simulink model "acc_RR_backup"  (R2021b)
settings: Solver=FixedStepAuto  StartTime=0.0  StopTime=40  FixedStep=0.0005  RelTol=1e-3
values from neighbouring files (symbols this model uses):
  s_path = [0 1.10508939428 2.2141958029 3.32141571172 4.42705301151 5.53154548532 6.63517443471 7.73808041313 8.84055018688 9.94289959674 11.0453539299 12.1480581097 ... (1001 elements, 1001x1)]    [200_100radius.mat]    (also in LV_Clothoid_S_Turn_path.mat = [0 0.966832089581 1.93621320584 2.90214024471 3.86476766313 ; NEDC_path.mat = [0 0.414605943146 0.832514087334 1.25401518562 1.68216660344; Straight_East_into_curve.mat = [0 1.65770560069 3.32192925577 4.98420060507 6.64484613518 8; acc_plot_backup.m = Station_HV_m)
  X_path = [0 1.10508939428 2.2141958029 3.32141571172 4.42705301151 5.53154548532 6.63517443471 7.73808041313 8.84055018688 9.94289959674 11.0453539299 12.1480581097 ... (1001 elements, 1001x1)]    [200_100radius.mat]    (also in LV_Clothoid_S_Turn_path.mat = [-10 -9.03316791042 -8.06378679416 -7.09785975529 -6.1352323; NEDC_path.mat = [0 0.414605943146 0.832514087334 1.25401518562 1.68216660344; Straight_East_into_curve.mat = [0 1.65770560069 3.32192925577 4.98420060507 6.64484613518 8; acc_plot_backup.m = X_HV_m)
  Y_path = [0 -1.70364610795e-18 -7.41532896709e-18 1.46822109542e-17 4.74557362791e-17 6.12980216762e-17 9.25043977736e-17 1.24088240159e-16 1.5099156923e-16 1.7058517853e-16 1.90629227614e-16 2.09673434424e-16 ... (1001 elements, 1001x1)]    [200_100radius.mat]    (also in LV_Clothoid_S_Turn_path.mat = [0 -8.46153035536e-19 5.07382551045e-18 2.07356032218e-17 3.; NEDC_path.mat = [0 -3.50680326162e-18 -2.14111304971e-18 3.38197671014e-18 3; Straight_East_into_curve.mat = [0 1.29197709199e-18 2.81882429322e-18 3.49020462564e-17 6.7; acc_plot_backup.m = Y_HV_m)
undefined symbols (not defined in the file or in its folder): C_TICK_TIME_S, ENUM_ACCSTATE_DISABLED, ENUM_ACCSTATE_OFF, ENUM_ACCSTATE_STANDBY, FALSE, KVDI_ACCLongPressTime_ms, KVDI_ACCMaxActSpeed_kph, KVDI_ACCSetSpdIntial_kph, KVDI_ACCSpdLargeChange_kph, KVDI_LongPressConTime_ms, ONE_FLOAT, ONE_INT, R, Rw, T, TRUE, ZERO_FLOAT, ZERO_INT
libraries: simulink x15, simulink_extras x2, Solver_SF x1
(part 2 of 4)

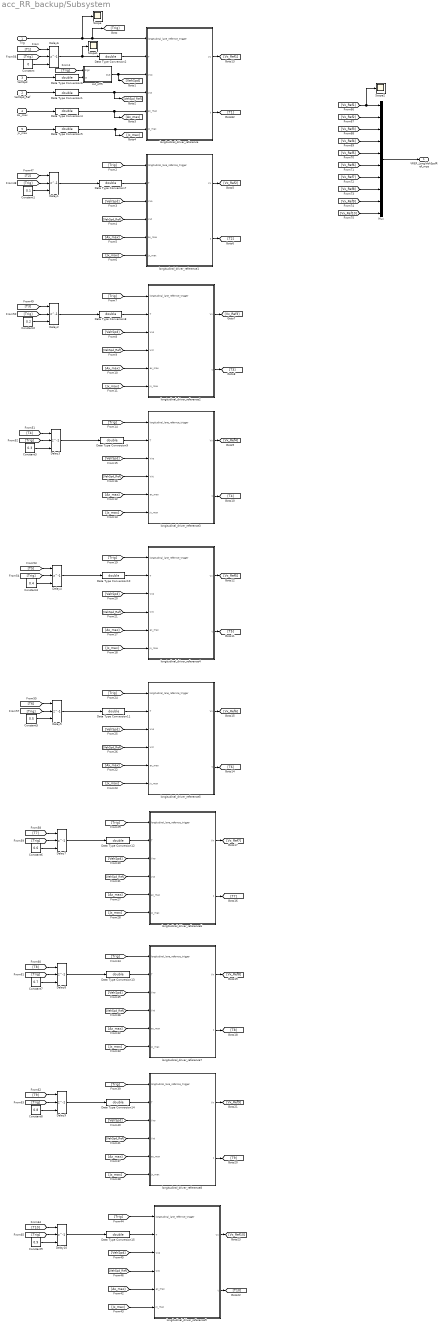
== system acc_RR_backup/Subsystem ==
  "Trig " : Inport
  VehSpd_Ref : Inport  Port=2
  VehSpd : Inport  Port=3
  Ax_max : Inport  Port=4
  Jx_max : Inport  Port=5
  Constant : Constant  Value=0
  Constant1 : Constant  Value=0.1
  Constant2 : Constant  Value=0.2
  Constant3 : Constant  Value=0.3
  Constant4 : Constant  Value=0.4
  Constant5 : Constant  Value=0.5
  Constant6 : Constant  Value=0.6
  Constant7 : Constant  Value=0.7
  Constant8 : Constant  Value=0.8
  Constant9 : Constant  Value=0.9
  Data Type Conversion{1..2,4..15} (14 alike) : DataTypeConversion  OutDataTypeStr=double
  Delay{1..10} (10 alike) : Delay  DelayLength=1  InitialConditionSource=Input port  ExternalReset=Rising
      settings: InputPortMap=u0,r5,p4
  Mux : Mux  Inputs=10
  Scope : Scope
  Scope1 : Scope
  Scope2 : Scope
  cut_off5 : Subsystem
  longitudinal_driver_reference : MATLAB Function  TreatAsAtomicUnit=on
  longitudinal_driver_reference1 : MATLAB Function  TreatAsAtomicUnit=on
  longitudinal_driver_reference2 : MATLAB Function  TreatAsAtomicUnit=on
  longitudinal_driver_reference3 : MATLAB Function  TreatAsAtomicUnit=on
  longitudinal_driver_reference4 : MATLAB Function  TreatAsAtomicUnit=on
  longitudinal_driver_reference5 : MATLAB Function  TreatAsAtomicUnit=on
  longitudinal_driver_reference6 : MATLAB Function  TreatAsAtomicUnit=on
  longitudinal_driver_reference7 : MATLAB Function  TreatAsAtomicUnit=on
  longitudinal_driver_reference8 : MATLAB Function  TreatAsAtomicUnit=on
  longitudinal_driver_reference9 : MATLAB Function  TreatAsAtomicUnit=on
  "VREF_LongiVehSpdRef_mps " : Outport
  wires:
  longitudinal_driver_reference/1(Vx) -> [Vx_Ref1]
  Mux/1 -> "VREF_LongiVehSpdRef_mps "/1
  Constant/1 -> Delay6/3
  [T1] -> Delay6/1
  Ax_max/1 -> Data Type Conversion4/1
  Jx_max/1 -> Data Type Conversion5/1
  VehSpd_Ref/1 -> Data Type Conversion1/1
  longitudinal_driver_reference/2(t) -> [T1]
  Delay6/1 -> Scope1/1, Data Type Conversion2/1
  [Trig] -> Delay6/2
  "Trig "/1 -> Scope/1, [Trig], longitudinal_driver_reference/1(longitudinal_lane_refernce_trigger)
  Data Type Conversion2/1 -> longitudinal_driver_reference/2(T)
  VehSpd/1 -> Data Type Conversion6/1
  Data Type Conversion1/1 -> [VehSpd_Ref], longitudinal_driver_reference/4(Vxt)
  cut_off5/1(Out) -> [VehSpd], longitudinal_driver_reference/3(Vxo)
  Data Type Conversion6/1 -> cut_off5/2(in)
  [Trig] -> cut_off5/1(sign)
  Data Type Conversion5/1 -> [Jx_max], longitudinal_driver_reference/6(jx_max)
  Data Type Conversion4/1 -> [Ax_max], longitudinal_driver_reference/5(ax_max)
  [Trig] -> longitudinal_driver_reference1/1(longitudinal_lane_refernce_trigger)
  [VehSpd] -> longitudinal_driver_reference1/3(Vxo)
  [VehSpd_Ref] -> longitudinal_driver_reference1/4(Vxt)
  [Ax_max] -> longitudinal_driver_reference1/5(ax_max)
  [Jx_max] -> longitudinal_driver_reference1/6(jx_max)
  [Jx_max] -> longitudinal_driver_reference2/6(jx_max)
  [Ax_max] -> longitudinal_driver_reference2/5(ax_max)
  [VehSpd_Ref] -> longitudinal_driver_reference2/4(Vxt)
  [VehSpd] -> longitudinal_driver_reference2/3(Vxo)
  [Trig] -> longitudinal_driver_reference2/1(longitudinal_lane_refernce_trigger)
  [Trig] -> longitudinal_driver_reference3/1(longitudinal_lane_refernce_trigger)
  [VehSpd] -> longitudinal_driver_reference3/3(Vxo)
  [VehSpd_Ref] -> longitudinal_driver_reference3/4(Vxt)
  [Ax_max] -> longitudinal_driver_reference3/5(ax_max)
  [Jx_max] -> longitudinal_driver_reference3/6(jx_max)
  [Jx_max] -> longitudinal_driver_reference4/6(jx_max)
  [Ax_max] -> longitudinal_driver_reference4/5(ax_max)
  [VehSpd_Ref] -> longitudinal_driver_reference4/4(Vxt)
  [VehSpd] -> longitudinal_driver_reference4/3(Vxo)
  [Trig] -> longitudinal_driver_reference4/1(longitudinal_lane_refernce_trigger)
  [Trig] -> longitudinal_driver_reference5/1(longitudinal_lane_refernce_trigger)
  [VehSpd] -> longitudinal_driver_reference5/3(Vxo)
  [VehSpd_Ref] -> longitudinal_driver_reference5/4(Vxt)
  [Ax_max] -> longitudinal_driver_reference5/5(ax_max)
  [Jx_max] -> longitudinal_driver_reference5/6(jx_max)
  [Jx_max] -> longitudinal_driver_reference6/6(jx_max)
  [Ax_max] -> longitudinal_driver_reference6/5(ax_max)
  [VehSpd_Ref] -> longitudinal_driver_reference6/4(Vxt)
  [VehSpd] -> longitudinal_driver_reference6/3(Vxo)
  [Trig] -> longitudinal_driver_reference6/1(longitudinal_lane_refernce_trigger)
  [Trig] -> longitudinal_driver_reference7/1(longitudinal_lane_refernce_trigger)
  [VehSpd] -> longitudinal_driver_reference7/3(Vxo)
  [VehSpd_Ref] -> longitudinal_driver_reference7/4(Vxt)
  [Ax_max] -> longitudinal_driver_reference7/5(ax_max)
  [Jx_max] -> longitudinal_driver_reference7/6(jx_max)
  [Jx_max] -> longitudinal_driver_reference8/6(jx_max)
  [Ax_max] -> longitudinal_driver_reference8/5(ax_max)
  [VehSpd_Ref] -> longitudinal_driver_reference8/4(Vxt)
  [VehSpd] -> longitudinal_driver_reference8/3(Vxo)
  [Trig] -> longitudinal_driver_reference8/1(longitudinal_lane_refernce_trigger)
  [Trig] -> longitudinal_driver_reference9/1(longitudinal_lane_refernce_trigger)
  [VehSpd] -> longitudinal_driver_reference9/3(Vxo)
  [VehSpd_Ref] -> longitudinal_driver_reference9/4(Vxt)
  [Ax_max] -> longitudinal_driver_reference9/5(ax_max)
  [Jx_max] -> longitudinal_driver_reference9/6(jx_max)
  longitudinal_driver_reference1/1(Vx) -> [Vx_Ref2]
  longitudinal_driver_reference1/2(t) -> [T2]
  [Trig] -> Delay1/2
  Delay1/1 -> Data Type Conversion7/1
  [T2] -> Delay1/1
  Data Type Conversion7/1 -> longitudinal_driver_reference1/2(T)
  Constant1/1 -> Delay1/3
  Constant2/1 -> Delay2/3
  Data Type Conversion8/1 -> longitudinal_driver_reference2/2(T)
  [T3] -> Delay2/1
  Delay2/1 -> Data Type Conversion8/1
  [Trig] -> Delay2/2
  longitudinal_driver_reference2/2(t) -> [T3]
  longitudinal_driver_reference2/1(Vx) -> [Vx_Ref3]
  [Trig] -> Delay3/2
  Delay3/1 -> Data Type Conversion9/1
  [T4] -> Delay3/1
  Data Type Conversion9/1 -> longitudinal_driver_reference3/2(T)
  Constant3/1 -> Delay3/3
  longitudinal_driver_reference3/1(Vx) -> [Vx_Ref4]
  longitudinal_driver_reference3/2(t) -> [T4]
  Constant4/1 -> Delay4/3
  Data Type Conversion10/1 -> longitudinal_driver_reference4/2(T)
  [T5] -> Delay4/1
  Delay4/1 -> Data Type Conversion10/1
  [Trig] -> Delay4/2
  longitudinal_driver_reference4/2(t) -> [T5]
  longitudinal_driver_reference4/1(Vx) -> [Vx_Ref5]
  longitudinal_driver_reference5/1(Vx) -> [Vx_Ref6]
  longitudinal_driver_reference5/2(t) -> [T6]
  [Trig] -> Delay5/2
  Delay5/1 -> Data Type Conversion11/1
  [T6] -> Delay5/1
  Constant5/1 -> Delay5/3
  Data Type Conversion11/1 -> longitudinal_driver_reference5/2(T)
  longitudinal_driver_reference6/2(t) -> [T7]
  longitudinal_driver_reference6/1(Vx) -> [Vx_Ref7]
  Constant6/1 -> Delay7/3
  [T7] -> Delay7/1
  Delay7/1 -> Data Type Conversion12/1
  [Trig] -> Delay7/2
  Data Type Conversion12/1 -> longitudinal_driver_reference6/2(T)
  [Trig] -> Delay8/2
  Delay8/1 -> Data Type Conversion13/1
  [T8] -> Delay8/1
  Constant7/1 -> Delay8/3
  Data Type Conversion13/1 -> longitudinal_driver_reference7/2(T)
  longitudinal_driver_reference7/1(Vx) -> [Vx_Ref8]
  longitudinal_driver_reference7/2(t) -> [T8]
  longitudinal_driver_reference8/2(t) -> [T9]
  longitudinal_driver_reference8/1(Vx) -> [Vx_Ref9]
  Data Type Conversion14/1 -> longitudinal_driver_reference8/2(T)
  Constant8/1 -> Delay9/3
  [T9] -> Delay9/1
  Delay9/1 -> Data Type Conversion14/1
  [Trig] -> Delay9/2
  longitudinal_driver_reference9/1(Vx) -> [Vx_Ref10]
  longitudinal_driver_reference9/2(t) -> [T10]
  [Trig] -> Delay10/2
  Delay10/1 -> Data Type Conversion15/1
  [T10] -> Delay10/1
  Constant9/1 -> Delay10/3
  Data Type Conversion15/1 -> longitudinal_driver_reference9/2(T)
  [Vx_Ref1] -> Scope2/1, Mux/1
  [Vx_Ref2] -> Mux/2
  [Vx_Ref3] -> Mux/3
  [Vx_Ref4] -> Mux/4
  [Vx_Ref5] -> Mux/5
  [Vx_Ref6] -> Mux/6
  [Vx_Ref7] -> Mux/7
  [Vx_Ref8] -> Mux/8
  [Vx_Ref9] -> Mux/9
  [Vx_Ref10] -> Mux/10

== system acc_RR_backup/Subsystem1 ==
  In1 : Inport
  Constant117 : Constant  Value=single(1)  OutDataTypeStr=single
  Relational Operator : RelationalOperator  OutDataTypeStr=boolean  RndMeth=Simplest
  Saturation5 : Saturate  UpperLimit=inf  LowerLimit=40/3.6
  Switch7 : Switch  Criteria=u2 ~= 0
  Out1 : Outport
  wires:
  Relational Operator/1 -> Switch7/2
  In1/1 -> Relational Operator/1, Switch7/1
  Constant117/1 -> Relational Operator/2, Switch7/3
  Switch7/1 -> Out1/1

== system acc_RR_backup/Subsystem16 ==
  C0 : Inport
  C1 : Inport  Port=2
  "C2 " : Inport  Port=3
  C3 : Inport  Port=4
  PrediDis : Inport  Port=5
  Add30 : Sum  Inputs=++++
  Fcn : Fcn  Expr=(u)^3
  Product : Product
  Product1 : Product
  Product2 : Product
  Square : Math  Operator=square  SignedPower=on  RndMeth=Zero  SaturateOnIntegerOverflow=on
  LeftDis : Outport  VectorParamsAs1DForOutWhenUnconnected=off
  wires:
  PrediDis/1 -> [PrediDis]
  [PrediDis] -> Square/1
  Product/1 -> Add30/2
  Product1/1 -> Add30/3
  "C2 "/1 -> Product1/1
  [PrediDis] -> Product/2
  [PrediDis] -> Fcn/1
  Fcn/1 -> Product2/2
  Square/1 -> Product1/2
  C0/1 -> Add30/1
  Product2/1 -> Add30/4
  C1/1 -> Product/1
  Add30/1 -> LeftDis/1
  C3/1 -> Product2/1

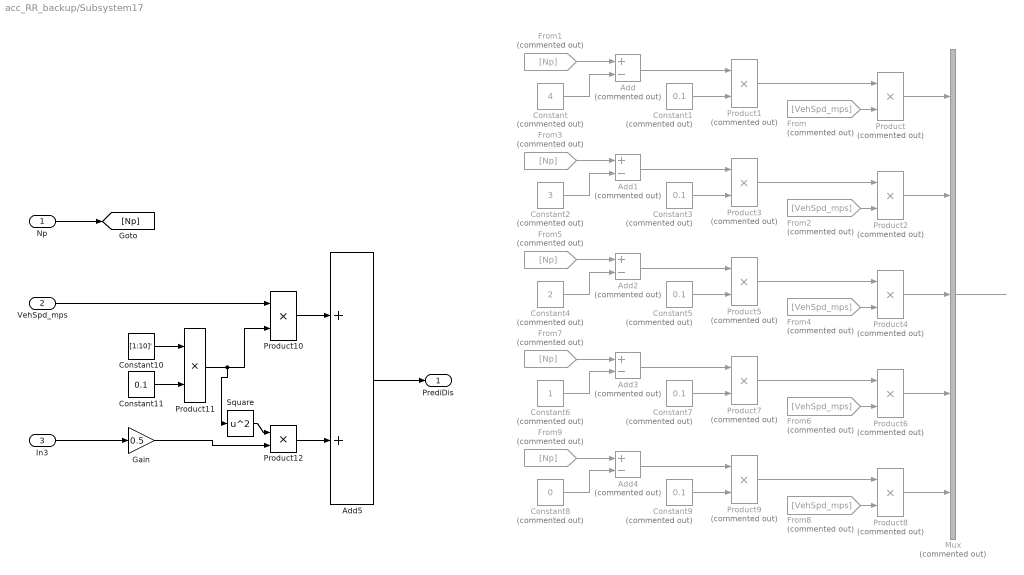
== system acc_RR_backup/Subsystem17 ==
  Np : Inport
  VehSpd_mps : Inport  Port=2
  In3 : Inport  Port=3
  Add{,1..4} (5 alike) : Sum  Commented=on  Inputs=+-
  Add5 : Sum
  Constant : Constant  Commented=on  Value=4
  Constant{1,3,5,7,9} (5 alike) : Constant  Commented=on  Value=0.1
  Constant10 : Constant  Value=[1:10]'
  Constant11 : Constant  Value=0.1
  Constant2 : Constant  Commented=on  Value=3
  Constant4 : Constant  Commented=on  Value=2
  Constant6 : Constant  Commented=on
  Constant8 : Constant  Commented=on  Value=0
  From{,2,4,6,8} (5 alike) : From  Commented=on  GotoTag=VehSpd_mps
  From{1,3,5,7,9} (5 alike) : From  Commented=on  GotoTag=Np
  Gain : Gain  Gain=0.5
  Mux : Mux  Commented=on  Inputs=5
  Product{,1..9} (10 alike) : Product  Commented=on
  Product10 : Product
  Product11 : Product
  Product12 : Product
  Square : Math  Operator=square  SaturateOnIntegerOverflow=on
  PrediDis : Outport  VectorParamsAs1DForOutWhenUnconnected=off
  wires:
  Product8/1 -> Mux/5
  Constant9/1 -> Product9/2
  Constant8/1 -> Add4/2
  From9/1 -> Add4/1
  Add4/1 -> Product9/1
  Product9/1 -> Product8/1
  From8/1 -> Product8/2
  From6/1 -> Product6/2
  Product7/1 -> Product6/1
  Add3/1 -> Product7/1
  From7/1 -> Add3/1
  Constant6/1 -> Add3/2
  Constant7/1 -> Product7/2
  Product6/1 -> Mux/4
  Product4/1 -> Mux/3
  Constant5/1 -> Product5/2
  Constant4/1 -> Add2/2
  From5/1 -> Add2/1
  Add2/1 -> Product5/1
  Product5/1 -> Product4/1
  From4/1 -> Product4/2
  Product2/1 -> Mux/2
  From2/1 -> Product2/2
  Product3/1 -> Product2/1
  Add1/1 -> Product3/1
  From3/1 -> Add1/1
  Constant2/1 -> Add1/2
  Constant3/1 -> Product3/2
  Constant1/1 -> Product1/2
  Constant/1 -> Add/2
  From1/1 -> Add/1
  Add/1 -> Product1/1
  Product1/1 -> Product/1
  From/1 -> Product/2
  Product/1 -> Mux/1
  Np/1 -> [Np]
  Mux/1 -> ?
  Product10/1 -> Add5/1
  VehSpd_mps/1 -> Product10/1
  Product11/1 -> Product10/2, Square/1
  Constant10/1 -> Product11/1
  Constant11/1 -> Product11/2
  Add5/1 -> PrediDis/1
  In3/1 -> Gain/1
  Product12/1 -> Add5/2
  Square/1 -> Product12/1
  Gain/1 -> Product12/2

== system acc_RR_backup/Subsystem2 ==
  T_cmd : Inport
  Gain : Gain  Gain=-0.25
  Gain2 : Gain  Gain=1/250
  Gain3 : Gain  Gain=1/150
  Saturation1 : Saturate  UpperLimit=0  LowerLimit=-inf
  Smooth_Switch1 : Subsystem  Commented=on  mask{tau=0.3, IC=0, T=0.1}
      mask prompts: tau "Time constant"; T "Sample time"
      mask Display:
      | fprintf('Discrete first order \n\n')
      | fprintf(['tau=' num2str(tau) '    IC=' num2str(IC)])
  Transfer Fcn1 : TransferFcn  Denominator=[0.3 1]
  Transfer Fcn2 : TransferFcn  Denominator=[0.3 1]
  Pb_LF : Outport
  Pb_RF : Outport  Port=2
  Pb_RL : Outport  Port=3
  Pb_RR : Outport  Port=4
  wires:
  Transfer Fcn1/1 -> Pb_RR/1, Pb_RL/1
  Transfer Fcn2/1 -> Pb_RF/1, Pb_LF/1
  Gain3/1 -> Transfer Fcn1/1
  Gain2/1 -> Transfer Fcn2/1
  Gain/1 -> Gain2/1, Gain3/1
  Saturation1/1 -> Gain/1
  T_cmd/1 -> Saturation1/1

== system acc_RR_backup/Subsystem20 ==
  Rx : Inport
  Ry : Inport  Port=2
  RVx : Inport  Port=3
  RVy : Inport  Port=4
  MATLAB Function4 : MATLAB Function  TreatAsAtomicUnit=on
  MATLAB Function6 : MATLAB Function  TreatAsAtomicUnit=on
  Scope23 : Scope  NumInputPorts=4
  distance1 : Subsystem
  distance2 : Subsystem
  theta_min : Outport  VectorParamsAs1DForOutWhenUnconnected=off
  theta_max : Outport  Port=2  VectorParamsAs1DForOutWhenUnconnected=off
  Vectory_ang : Outport  Port=3  VectorParamsAs1DForOutWhenUnconnected=off
  wires:
  Rx/1 -> MATLAB Function6/1(Rx), MATLAB Function4/1(Rx)
  Ry/1 -> MATLAB Function6/2(Ry)
  MATLAB Function6/5(theta_min) -> theta_min/1
  RVx/1 -> MATLAB Function4/2(RVx)
  MATLAB Function6/2(theta_2) -> Scope23/2
  MATLAB Function6/4(theta_4) -> Scope23/4
  MATLAB Function6/1(theta_1) -> Scope23/1
  MATLAB Function6/3(theta_3) -> Scope23/3
  MATLAB Function6/6(theta_max) -> theta_max/1
  MATLAB Function4/1(ang) -> Vectory_ang/1
  RVy/1 -> MATLAB Function4/3(RVy)

== system acc_RR_backup/Subsystem3 ==
  Jerk : Inport
  Vx : Inport  Port=2
  Constant1 : Constant  Value=0  OutDataTypeStr=single
  Constant117 : Constant  Value=0.5  OutDataTypeStr=single
  Relational Operator : RelationalOperator  OutDataTypeStr=boolean  RndMeth=Simplest
  Switch7 : Switch  Criteria=u2 ~= 0
  Out1 : Outport
  wires:
  Relational Operator/1 -> Switch7/2
  Vx/1 -> Relational Operator/1
  Constant117/1 -> Relational Operator/2
  Switch7/1 -> Out1/1
  Constant1/1 -> Switch7/3
  Jerk/1 -> Switch7/1

== system acc_RR_backup/Subsystem4 ==
  new_value : Inport
  Constant44 : Constant  Value=0.25
  Constant48 : Constant  Value=0.1
  Delay1 : Delay  DelayLength=1  SampleTime=0.1
  rolling_avg1 : Subsystem
  new_ave : Outport
  wires:
  Constant44/1 -> rolling_avg1/4(tc)
  new_value/1 -> rolling_avg1/1(new_value)
  Constant48/1 -> rolling_avg1/3(delta_t)  "T"
  Delay1/1 -> rolling_avg1/2(old_ave)
  rolling_avg1/1(new_ave) -> new_ave/1, Delay1/1

== system acc_RR_backup/Subsystem5 ==
  new_value : Inport
  Constant44 : Constant  Value=0.3
  Constant48 : Constant  Value=0.1
  Delay1 : Delay  DelayLength=1  SampleTime=0.1
  rolling_avg1 : Subsystem
  new_ave : Outport
  wires:
  rolling_avg1/1(new_ave) -> Delay1/1, new_ave/1
  Delay1/1 -> rolling_avg1/2(old_ave)
  Constant48/1 -> rolling_avg1/3(delta_t)  "T"
  new_value/1 -> rolling_avg1/1(new_value)
  Constant44/1 -> rolling_avg1/4(tc)

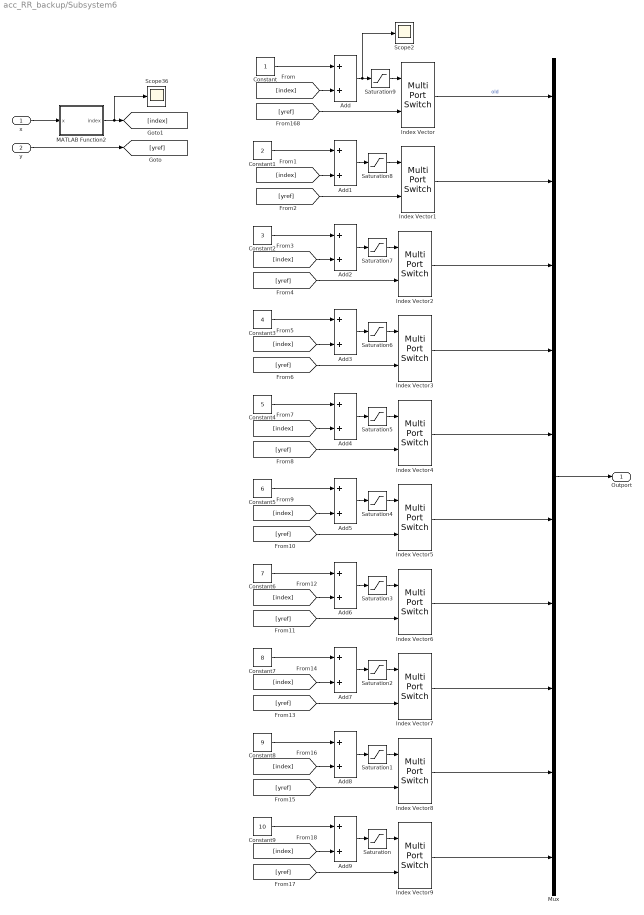
== system acc_RR_backup/Subsystem6 ==
  x : Inport
  y : Inport  Port=2
  Add{,1..9} (10 alike) : Sum
  Constant : Constant
  Constant1 : Constant  Value=2
  Constant2 : Constant  Value=3
  Constant3 : Constant  Value=4
  Constant4 : Constant  Value=5
  Constant5 : Constant  Value=6
  Constant6 : Constant  Value=7
  Constant7 : Constant  Value=8
  Constant8 : Constant  Value=9
  Constant9 : Constant  Value=10
  Index Vector{,1..9} (10 alike) : MultiPortSwitch  Inputs=1
  MATLAB Function2 : MATLAB Function  TreatAsAtomicUnit=on
  Mux : Mux  Inputs=10
  Saturation{,1..9} (10 alike) : Saturate  UpperLimit=30  LowerLimit=1
  Scope2 : Scope
  Scope36 : Scope
  Outport : Outport
  wires:
  Add/1 -> Scope2/1, Saturation9/1
  [yref] -> Index Vector/2
  MATLAB Function2/1(index) -> Scope36/1, [index]
  Index Vector/1 -> Mux/1  "old"
  x/1 -> MATLAB Function2/1(x)
  y/1 -> [yref]
  [index] -> Add/2
  Constant/1 -> Add/1
  Constant1/1 -> Add1/1
  [index] -> Add1/2
  [yref] -> Index Vector1/2
  Add1/1 -> Saturation8/1
  Add2/1 -> Saturation7/1
  [yref] -> Index Vector2/2
  [index] -> Add2/2
  Constant2/1 -> Add2/1
  Constant3/1 -> Add3/1
  [index] -> Add3/2
  [yref] -> Index Vector3/2
  Add3/1 -> Saturation6/1
  Add4/1 -> Saturation5/1
  [yref] -> Index Vector4/2
  [index] -> Add4/2
  Constant4/1 -> Add4/1
  Constant5/1 -> Add5/1
  [index] -> Add5/2
  [yref] -> Index Vector5/2
  Add5/1 -> Saturation4/1
  Add6/1 -> Saturation3/1
  [yref] -> Index Vector6/2
  [index] -> Add6/2
  Constant6/1 -> Add6/1
  Constant7/1 -> Add7/1
  [index] -> Add7/2
  [yref] -> Index Vector7/2
  Add7/1 -> Saturation2/1
  Add8/1 -> Saturation1/1
  [yref] -> Index Vector8/2
  [index] -> Add8/2
  Constant8/1 -> Add8/1
  Constant9/1 -> Add9/1
  [index] -> Add9/2
  [yref] -> Index Vector9/2
  Add9/1 -> Saturation/1
  Saturation/1 -> Index Vector9/1
  Saturation1/1 -> Index Vector8/1
  Saturation2/1 -> Index Vector7/1
  Saturation3/1 -> Index Vector6/1
  Saturation4/1 -> Index Vector5/1
  Saturation5/1 -> Index Vector4/1
  Saturation6/1 -> Index Vector3/1
  Saturation7/1 -> Index Vector2/1
  Saturation8/1 -> Index Vector1/1
  Saturation9/1 -> Index Vector/1
  Index Vector9/1 -> Mux/10
  Index Vector8/1 -> Mux/9
  Index Vector7/1 -> Mux/8
  Index Vector1/1 -> Mux/2
  Index Vector2/1 -> Mux/3
  Index Vector3/1 -> Mux/4
  Index Vector4/1 -> Mux/5
  Index Vector5/1 -> Mux/6
  Index Vector6/1 -> Mux/7
  Mux/1 -> Outport/1

== system acc_RR_backup/Subsystem7 ==
  Rx : Inport
  Ry : Inport  Port=2
  RVx : Inport  Port=3
  RVy : Inport  Port=4
  MATLAB Function4 : MATLAB Function  TreatAsAtomicUnit=on
  MATLAB Function6 : MATLAB Function  TreatAsAtomicUnit=on
  Scope23 : Scope  NumInputPorts=4
  distance1 : Subsystem
  distance2 : Subsystem
  theta_min : Outport  VectorParamsAs1DForOutWhenUnconnected=off
  theta_max : Outport  Port=2  VectorParamsAs1DForOutWhenUnconnected=off
  Vectory_ang : Outport  Port=3  VectorParamsAs1DForOutWhenUnconnected=off
  wires:
  RVy/1 -> MATLAB Function4/3(RVy)
  MATLAB Function4/1(ang) -> Vectory_ang/1
  MATLAB Function6/6(theta_max) -> theta_max/1
  MATLAB Function6/3(theta_3) -> Scope23/3
  MATLAB Function6/1(theta_1) -> Scope23/1
  MATLAB Function6/4(theta_4) -> Scope23/4
  MATLAB Function6/2(theta_2) -> Scope23/2
  RVx/1 -> MATLAB Function4/2(RVx)
  MATLAB Function6/5(theta_min) -> theta_min/1
  Ry/1 -> MATLAB Function6/2(Ry)
  Rx/1 -> MATLAB Function4/1(Rx), MATLAB Function6/1(Rx)

== system acc_RR_backup/Subsystem8 ==
  TTC : Inport
  Mode : Inport  Port=2
  Constant1 : Constant  Value=0
  Switch : Switch  Criteria=u2 ~= 0
  Out1 : Outport
  wires:
  Constant1/1 -> Switch/3
  TTC/1 -> Switch/1
  Switch/1 -> Out1/1
  Mode/1 -> Switch/2

== system acc_RR_backup/V_rel Estimation ==
  a_c : Inport
  S_rel : Inport  Port=2
  initial_value : Inport  Port=3
  Add3 : Sum  Inputs=-+
  Delay1 : Delay  DelayLength=1  InitialConditionSource=Input port  SampleTime=0.1
      settings: InputPortMap=u0,p4
  Kalman filter : Subsystem
  sample time : Gain  Gain=1/0.1
  s_rel : Outport
  v_rel : Outport  Port=2
  a_rel : Outport  Port=3
  wires:
  S_rel/1 -> Kalman filter/2(S_rel)
  Kalman filter/1(s_rel) -> s_rel/1
  Add3/1 -> sample time/1
  Delay1/1 -> Add3/1
  a_c/1 -> Delay1/1, Delay1/2, Add3/2
  Kalman filter/2(v_rel) -> v_rel/1
  sample time/1 -> Kalman filter/1(Jerk)  "Jerk"
  Kalman filter/3(a_rel) -> a_rel/1
  initial_value/1 -> Kalman filter/3(initial_value)

== system acc_RR_backup/acceleration_apr1 ==
  acc_b : Inport
  Abs : Abs
  Constant1 : Constant  Value=0
  Switch : Switch  Criteria=u2 > Threshold  Threshold=0.01
  acc_a : Outport  VectorParamsAs1DForOutWhenUnconnected=off
  wires:
  Switch/1 -> acc_a/1
  acc_b/1 -> Abs/1, Switch/1
  Constant1/1 -> Switch/3
  Abs/1 -> Switch/2

== system acc_RR_backup/acceleration_apr4 ==
  acc_b : Inport
  Abs : Abs
  Constant1 : Constant  Value=0
  Switch : Switch  Criteria=u2 > Threshold  Threshold=0.01
  acc_a : Outport  VectorParamsAs1DForOutWhenUnconnected=off
  wires:
  Abs/1 -> Switch/2
  Constant1/1 -> Switch/3
  acc_b/1 -> Switch/1, Abs/1
  Switch/1 -> acc_a/1

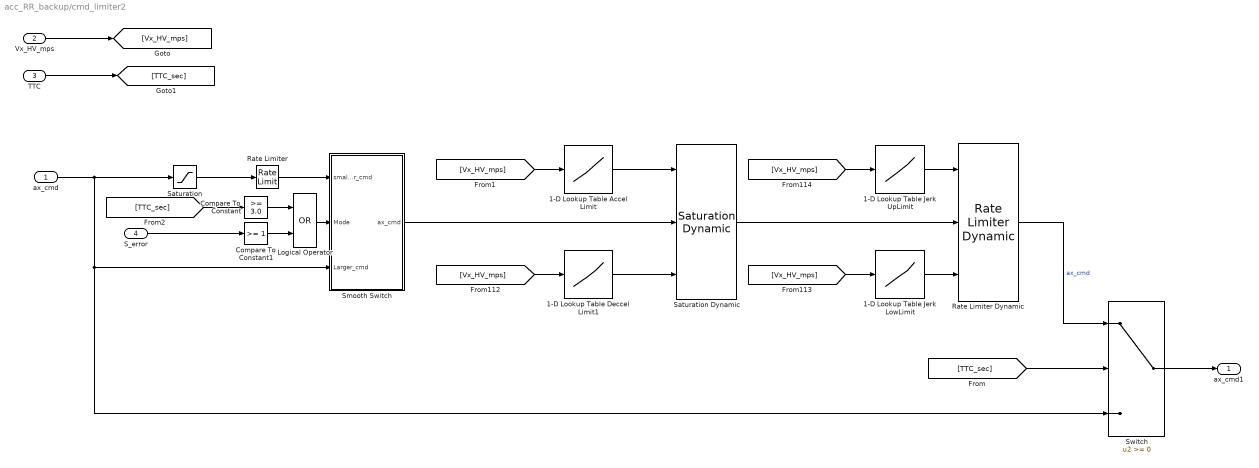
== system acc_RR_backup/cmd_limiter2 ==
  ax_cmd : Inport
  Vx_HV_mps : Inport  Port=2
  TTC : Inport  Port=3
  S_error : Inport  Port=4
  1-D Lookup Table Accel Limit : Lookup_n-D  NumberOfTableDimensions=1  BreakpointsForDimension1=[0,5,20,30]  Table=[4,4,2,2]  InternalRulePriority=Speed  RndMeth=Simplest  InputSameDT=on
  1-D Lookup Table Deccel Limit1 : Lookup_n-D  NumberOfTableDimensions=1  BreakpointsForDimension1=[0,5,20,30]  Table=[-5,-5,-2.5,-2.5]  InternalRulePriority=Speed  RndMeth=Simplest  InputSameDT=on
  1-D Lookup Table Jerk LowLimit : Lookup_n-D  NumberOfTableDimensions=1  BreakpointsForDimension1=[0,5,20,30]  Table=[-5,-5,-2.5,-2.5]  InternalRulePriority=Speed  RndMeth=Simplest  InputSameDT=on
  1-D Lookup Table Jerk UpLimit : Lookup_n-D  NumberOfTableDimensions=1  BreakpointsForDimension1=[0,5,20,30]  Table=[5,5,2.5,2.5]  InternalRulePriority=Speed  RndMeth=Simplest  InputSameDT=on
  Compare To Constant : simulink/Logic and Bit Operations/Compare To Constant  relop=>=  const=3.0  OutDataTypeStr=boolean
  Compare To Constant1 : simulink/Logic and Bit Operations/Compare To Constant  relop=>=  const=1  OutDataTypeStr=boolean
  Logical Operator : Logic  Operator=OR  AllPortsSameDT=off  OutDataTypeStr=boolean
  Rate Limiter : RateLimiter  RisingSlewLimit=2.5  FallingSlewLimit=-2.5  SampleTimeMode=inherited
  Rate Limiter Dynamic : simulink/Discontinuities/Rate Limiter Dynamic
  Saturation : Saturate  UpperLimit=2  LowerLimit=-2
  Saturation Dynamic : simulink/Discontinuities/Saturation Dynamic  OutMin=[]  OutMax=[]  OutDataTypeStr=Inherit: Same as second input  OutDataType=fixdt(1, 16)  OutScaling=2^-10  DoSatur=off
  Smooth Switch : Subsystem
  Switch : Switch
  ax_cmd1 : Outport
  wires:
  1-D Lookup Table Accel Limit/1 -> Saturation Dynamic/1
  [Vx_HV_mps] -> 1-D Lookup Table Jerk UpLimit/1
  1-D Lookup Table Jerk UpLimit/1 -> Rate Limiter Dynamic/1
  [Vx_HV_mps] -> 1-D Lookup Table Deccel Limit1/1
  [Vx_HV_mps] -> 1-D Lookup Table Jerk LowLimit/1
  1-D Lookup Table Deccel Limit1/1 -> Saturation Dynamic/3
  1-D Lookup Table Jerk LowLimit/1 -> Rate Limiter Dynamic/3
  Vx_HV_mps/1 -> [Vx_HV_mps]
  Saturation Dynamic/1 -> Rate Limiter Dynamic/2
  Rate Limiter Dynamic/1 -> Switch/1  "ax_cmd"
  [TTC_sec] -> Switch/2
  Switch/1 -> ax_cmd1/1
  TTC/1 -> [TTC_sec]
  Smooth Switch/1(ax_cmd) -> Saturation Dynamic/2
  [Vx_HV_mps] -> 1-D Lookup Table Accel Limit/1
  Saturation/1 -> Rate Limiter/1
  ax_cmd/1 -> Saturation/1, Switch/3, Smooth Switch/3(Larger_cmd)
  [TTC_sec] -> Compare To Constant/1
  Compare To Constant/1 -> Logical Operator/1
  Logical Operator/1 -> Smooth Switch/2(Mode)
  Compare To Constant1/1 -> Logical Operator/2
  S_error/1 -> Compare To Constant1/1
  Rate Limiter/1 -> Smooth Switch/1(smaller_cmd)

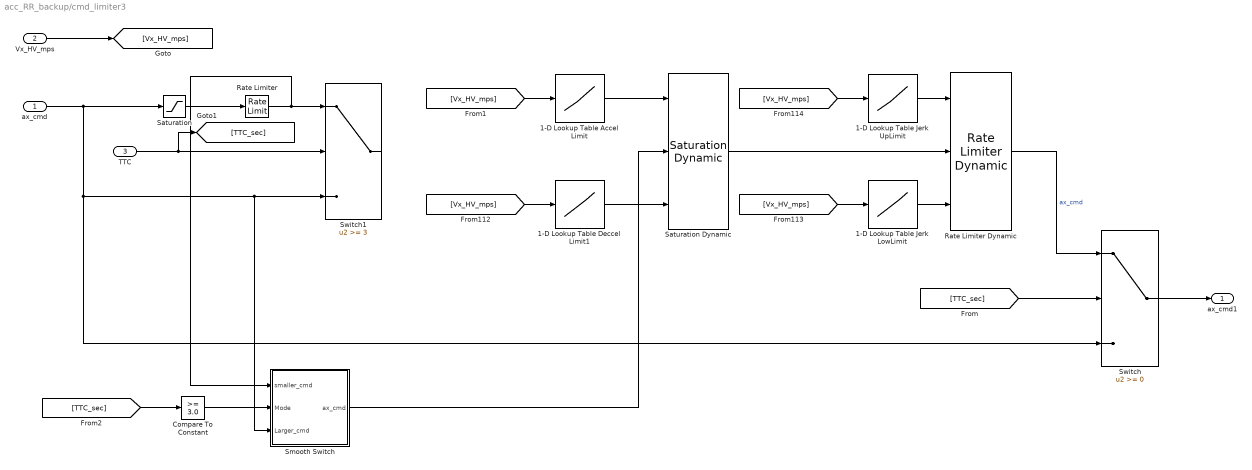
== system acc_RR_backup/cmd_limiter3 ==
  ax_cmd : Inport
  Vx_HV_mps : Inport  Port=2
  TTC : Inport  Port=3
  1-D Lookup Table Accel Limit : Lookup_n-D  NumberOfTableDimensions=1  BreakpointsForDimension1=[0,5,20,30]  Table=[4,4,2,2]  InternalRulePriority=Speed  RndMeth=Simplest  InputSameDT=on
  1-D Lookup Table Deccel Limit1 : Lookup_n-D  NumberOfTableDimensions=1  BreakpointsForDimension1=[0,5,20,30]  Table=[-5,-5,-2.5,-2.5]  InternalRulePriority=Speed  RndMeth=Simplest  InputSameDT=on
  1-D Lookup Table Jerk LowLimit : Lookup_n-D  NumberOfTableDimensions=1  BreakpointsForDimension1=[0,5,20,30]  Table=[-5,-5,-2.5,-2.5]  InternalRulePriority=Speed  RndMeth=Simplest  InputSameDT=on
  1-D Lookup Table Jerk UpLimit : Lookup_n-D  NumberOfTableDimensions=1  BreakpointsForDimension1=[0,5,20,30]  Table=[5,5,2.5,2.5]  InternalRulePriority=Speed  RndMeth=Simplest  InputSameDT=on
  Compare To Constant : simulink/Logic and Bit Operations/Compare To Constant  relop=>=  const=3.0  OutDataTypeStr=boolean
  Rate Limiter : RateLimiter  RisingSlewLimit=2.5  FallingSlewLimit=-2.5  SampleTimeMode=inherited
  Rate Limiter Dynamic : simulink/Discontinuities/Rate Limiter Dynamic
  Saturation : Saturate  UpperLimit=2  LowerLimit=-2
  Saturation Dynamic : simulink/Discontinuities/Saturation Dynamic  OutMin=[]  OutMax=[]  OutDataTypeStr=Inherit: Same as second input  OutDataType=fixdt(1, 16)  OutScaling=2^-10  DoSatur=off
  Smooth Switch : Subsystem
  Switch : Switch
  Switch1 : Switch  Threshold=3
  ax_cmd1 : Outport
  wires:
  Compare To Constant/1 -> Smooth Switch/2(Mode)
  [TTC_sec] -> Compare To Constant/1
  Rate Limiter/1 -> Switch1/1, Smooth Switch/1(smaller_cmd)
  Saturation/1 -> Rate Limiter/1
  [Vx_HV_mps] -> 1-D Lookup Table Accel Limit/1
  Smooth Switch/1(ax_cmd) -> Saturation Dynamic/2
  TTC/1 -> [TTC_sec], Switch1/2
  Switch/1 -> ax_cmd1/1
  [TTC_sec] -> Switch/2
  Rate Limiter Dynamic/1 -> Switch/1  "ax_cmd"
  ax_cmd/1 -> Switch/3, Switch1/3, Smooth Switch/3(Larger_cmd), Saturation/1
  Saturation Dynamic/1 -> Rate Limiter Dynamic/2
  Vx_HV_mps/1 -> [Vx_HV_mps]
  1-D Lookup Table Jerk LowLimit/1 -> Rate Limiter Dynamic/3
  1-D Lookup Table Deccel Limit1/1 -> Saturation Dynamic/3
  [Vx_HV_mps] -> 1-D Lookup Table Jerk LowLimit/1
  [Vx_HV_mps] -> 1-D Lookup Table Deccel Limit1/1
  1-D Lookup Table Jerk UpLimit/1 -> Rate Limiter Dynamic/1
  [Vx_HV_mps] -> 1-D Lookup Table Jerk UpLimit/1
  1-D Lookup Table Accel Limit/1 -> Saturation Dynamic/1

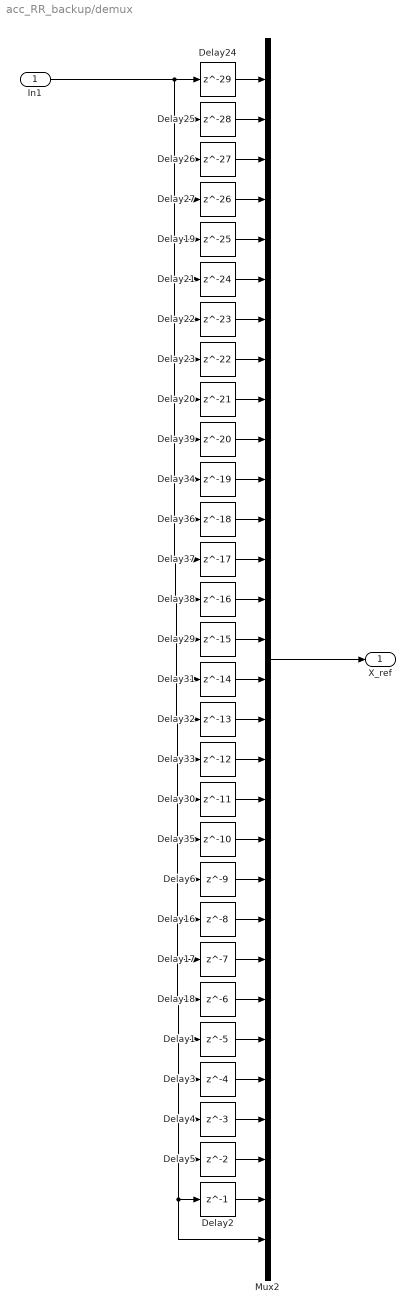
== system acc_RR_backup/demux ==
  In1 : Inport
  Delay1 : Delay  DelayLength=5
  Delay16 : Delay  DelayLength=8
  Delay17 : Delay  DelayLength=7
  Delay18 : Delay  DelayLength=6
  Delay19 : Delay  DelayLength=25
  Delay2 : Delay  DelayLength=1
  Delay20 : Delay  DelayLength=21
  Delay21 : Delay  DelayLength=24
  Delay22 : Delay  DelayLength=23
  Delay23 : Delay  DelayLength=22
  Delay24 : Delay  DelayLength=29
  Delay25 : Delay  DelayLength=28
  Delay26 : Delay  DelayLength=27
  Delay27 : Delay  DelayLength=26
  Delay29 : Delay  DelayLength=15
  Delay3 : Delay  DelayLength=4
  Delay30 : Delay  DelayLength=11
  Delay31 : Delay  DelayLength=14
  Delay32 : Delay  DelayLength=13
  Delay33 : Delay  DelayLength=12
  Delay34 : Delay  DelayLength=19
  Delay35 : Delay  DelayLength=10
  Delay36 : Delay  DelayLength=18
  Delay37 : Delay  DelayLength=17
  Delay38 : Delay  DelayLength=16
  Delay39 : Delay  DelayLength=20
  Delay4 : Delay  DelayLength=3
  Delay5 : Delay
  Delay6 : Delay  DelayLength=9
  Mux2 : Mux  Inputs=30
  X_ref : Outport
  wires:
  Delay24/1 -> Mux2/1
  In1/1 -> Delay22/1, Delay23/1, Delay30/1, Mux2/30, Delay2/1, Delay5/1, Delay4/1, Delay3/1, Delay1/1, Delay18/1, Delay17/1, Delay16/1, Delay6/1, Delay35/1, Delay33/1, Delay32/1, Delay31/1, Delay29/1, Delay38/1, Delay37/1, Delay36/1, Delay34/1, Delay39/1, Delay20/1, Delay21/1, Delay19/1, Delay27/1, Delay26/1, Delay25/1, Delay24/1
  Delay26/1 -> Mux2/3
  Delay23/1 -> Mux2/8
  Delay20/1 -> Mux2/9
  Delay25/1 -> Mux2/2
  Delay22/1 -> Mux2/7
  Delay21/1 -> Mux2/6
  Delay27/1 -> Mux2/4
  Delay19/1 -> Mux2/5
  Delay2/1 -> Mux2/29
  Delay5/1 -> Mux2/28
  Delay4/1 -> Mux2/27
  Delay3/1 -> Mux2/26
  Delay1/1 -> Mux2/25
  Delay18/1 -> Mux2/24
  Delay17/1 -> Mux2/23
  Delay16/1 -> Mux2/22
  Delay6/1 -> Mux2/21
  Delay35/1 -> Mux2/20
  Delay30/1 -> Mux2/19
  Delay33/1 -> Mux2/18
  Delay32/1 -> Mux2/17
  Delay34/1 -> Mux2/11
  Delay36/1 -> Mux2/12
  Delay37/1 -> Mux2/13
  Delay38/1 -> Mux2/14
  Delay29/1 -> Mux2/15
  Delay31/1 -> Mux2/16
  Delay39/1 -> Mux2/10
  Mux2/1 -> X_ref/1

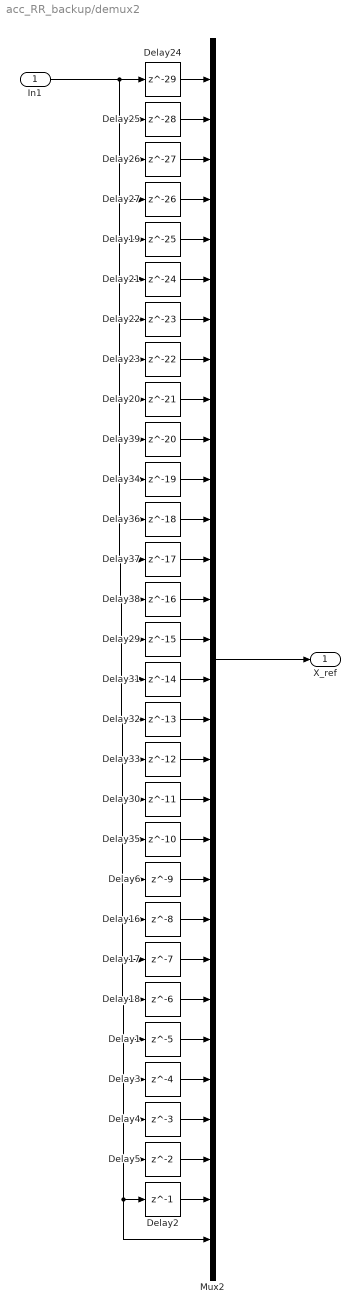
== system acc_RR_backup/demux2 ==
  In1 : Inport
  Delay1 : Delay  DelayLength=5
  Delay16 : Delay  DelayLength=8
  Delay17 : Delay  DelayLength=7
  Delay18 : Delay  DelayLength=6
  Delay19 : Delay  DelayLength=25
  Delay2 : Delay  DelayLength=1
  Delay20 : Delay  DelayLength=21
  Delay21 : Delay  DelayLength=24
  Delay22 : Delay  DelayLength=23
  Delay23 : Delay  DelayLength=22
  Delay24 : Delay  DelayLength=29
  Delay25 : Delay  DelayLength=28
  Delay26 : Delay  DelayLength=27
  Delay27 : Delay  DelayLength=26
  Delay29 : Delay  DelayLength=15
  Delay3 : Delay  DelayLength=4
  Delay30 : Delay  DelayLength=11
  Delay31 : Delay  DelayLength=14
  Delay32 : Delay  DelayLength=13
  Delay33 : Delay  DelayLength=12
  Delay34 : Delay  DelayLength=19
  Delay35 : Delay  DelayLength=10
  Delay36 : Delay  DelayLength=18
  Delay37 : Delay  DelayLength=17
  Delay38 : Delay  DelayLength=16
  Delay39 : Delay  DelayLength=20
  Delay4 : Delay  DelayLength=3
  Delay5 : Delay
  Delay6 : Delay  DelayLength=9
  Mux2 : Mux  Inputs=30
  X_ref : Outport
  wires:
  Mux2/1 -> X_ref/1
  Delay39/1 -> Mux2/10
  Delay31/1 -> Mux2/16
  Delay29/1 -> Mux2/15
  Delay38/1 -> Mux2/14
  Delay37/1 -> Mux2/13
  Delay36/1 -> Mux2/12
  Delay34/1 -> Mux2/11
  Delay32/1 -> Mux2/17
  Delay33/1 -> Mux2/18
  Delay30/1 -> Mux2/19
  Delay35/1 -> Mux2/20
  Delay6/1 -> Mux2/21
  Delay16/1 -> Mux2/22
  Delay17/1 -> Mux2/23
  Delay18/1 -> Mux2/24
  Delay1/1 -> Mux2/25
  Delay3/1 -> Mux2/26
  Delay4/1 -> Mux2/27
  Delay5/1 -> Mux2/28
  Delay2/1 -> Mux2/29
  Delay19/1 -> Mux2/5
  Delay27/1 -> Mux2/4
  Delay21/1 -> Mux2/6
  Delay22/1 -> Mux2/7
  Delay25/1 -> Mux2/2
  Delay20/1 -> Mux2/9
  Delay23/1 -> Mux2/8
  Delay26/1 -> Mux2/3
  In1/1 -> Delay24/1, Delay25/1, Delay26/1, Delay27/1, Delay19/1, Delay21/1, Delay20/1, Delay39/1, Delay34/1, Delay36/1, Delay37/1, Delay38/1, Delay29/1, Delay31/1, Delay32/1, Delay33/1, Delay35/1, Delay6/1, Delay16/1, Delay17/1, Delay18/1, Delay1/1, Delay3/1, Delay4/1, Delay5/1, Delay2/1, Mux2/30, Delay30/1, Delay23/1, Delay22/1
  Delay24/1 -> Mux2/1

== system acc_RR_backup/divide ==
  dividend : Inport
  divisor : Inport  Port=2
  default_value : Inport  Port=3
  Divide : Product  Inputs=*/
  Interval Test : simulink/Logic and Bit Operations/Interval Test  IntervalClosedRight=on  uplimit=1  IntervalClosedLeft=on  lowlimit=-1  OutDataTypeStr=boolean
  Logical Operator : Logic  Operator=NOT  Inputs=1  AllPortsSameDT=off  OutDataTypeStr=boolean
  Scope : Scope
  Switch : Switch  Criteria=u2 ~= 0  Threshold=0.5
  quotient : Outport
  wires:
  Logical Operator/1 -> Switch/2
  default_value/1 -> Switch/3  "default_value"
  Interval Test/1 -> Scope/1, Logical Operator/1
  Switch/1 -> quotient/1
  Divide/1 -> Switch/1
  divisor/1 -> Interval Test/1, Divide/2  "divisor"
  dividend/1 -> Divide/1  "dividend"

== system acc_RR_backup/divide1 ==
  dividend : Inport
  divisor : Inport  Port=2
  default_value : Inport  Port=3
  Divide : Product  Inputs=*/
  Interval Test : simulink/Logic and Bit Operations/Interval Test  IntervalClosedRight=on  uplimit=1  IntervalClosedLeft=on  lowlimit=-1  OutDataTypeStr=boolean
  Logical Operator : Logic  Operator=NOT  Inputs=1  AllPortsSameDT=off  OutDataTypeStr=boolean
  Scope : Scope
  Switch : Switch  Criteria=u2 ~= 0  Threshold=0.5
  quotient : Outport
  wires:
  Logical Operator/1 -> Switch/2
  default_value/1 -> Switch/3  "default_value"
  Interval Test/1 -> Scope/1, Logical Operator/1
  Switch/1 -> quotient/1
  Divide/1 -> Switch/1
  divisor/1 -> Interval Test/1, Divide/2  "divisor"
  dividend/1 -> Divide/1  "dividend"

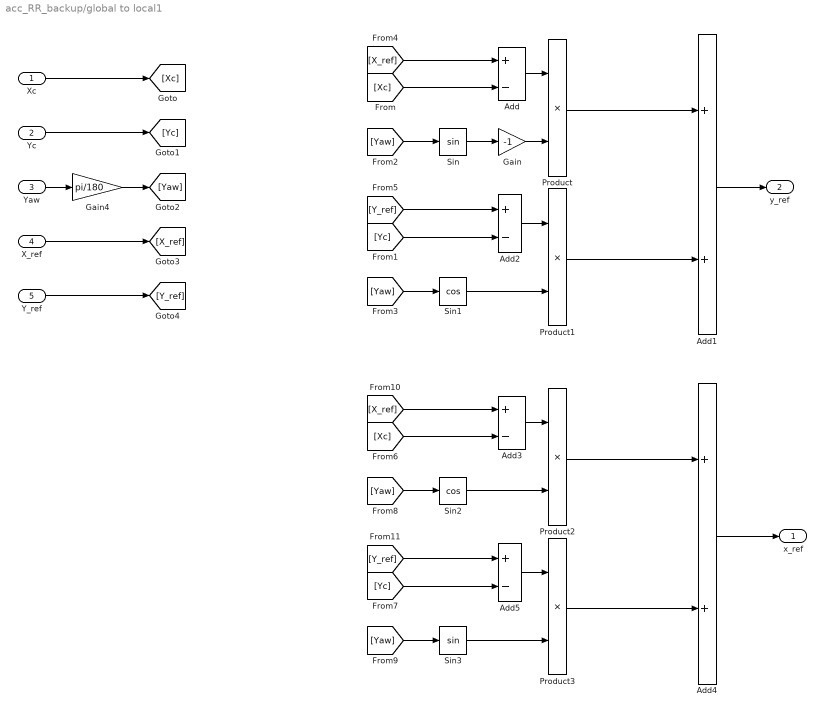
== system acc_RR_backup/global to local1 ==
  Xc : Inport
  Yc : Inport  Port=2
  Yaw : Inport  Port=3
  X_ref : Inport  Port=4
  Y_ref : Inport  Port=5
  Add{,2..3,5} (4 alike) : Sum  Inputs=+-
  Add1 : Sum
  Add4 : Sum
  Gain : Gain  Gain=-1
  Gain4 : Gain  Gain=pi/180
  Product{,1..3} (4 alike) : Product
  Sin : Trigonometry
  Sin1 : Trigonometry  Operator=cos
  Sin2 : Trigonometry  Operator=cos
  Sin3 : Trigonometry
  x_ref : Outport
  y_ref : Outport  Port=2
  wires:
  [X_ref] -> Add/1
  [Y_ref] -> Add2/1
  Sin/1 -> Gain/1
  Gain/1 -> Product/2
  Add/1 -> Product/1
  Product/1 -> Add1/1
  Sin1/1 -> Product1/2
  Add2/1 -> Product1/1
  Product1/1 -> Add1/2
  Add1/1 -> y_ref/1
  [Yaw] -> Sin/1
  [Yc] -> Add2/2
  [Xc] -> Add/2
  Xc/1 -> [Xc]
  Yc/1 -> [Yc]
  Yaw/1 -> Gain4/1
  [Yaw] -> Sin1/1
  X_ref/1 -> [X_ref]
  Y_ref/1 -> [Y_ref]
  Gain4/1 -> [Yaw]
  [Yaw] -> Sin3/1
  [Xc] -> Add3/2
  [Yc] -> Add5/2
  [Yaw] -> Sin2/1
  Add4/1 -> x_ref/1
  Product3/1 -> Add4/2
  Add5/1 -> Product3/1
  Sin3/1 -> Product3/2
  Product2/1 -> Add4/1
  Add3/1 -> Product2/1
  Sin2/1 -> Product2/2
  [Y_ref] -> Add5/1
  [X_ref] -> Add3/1

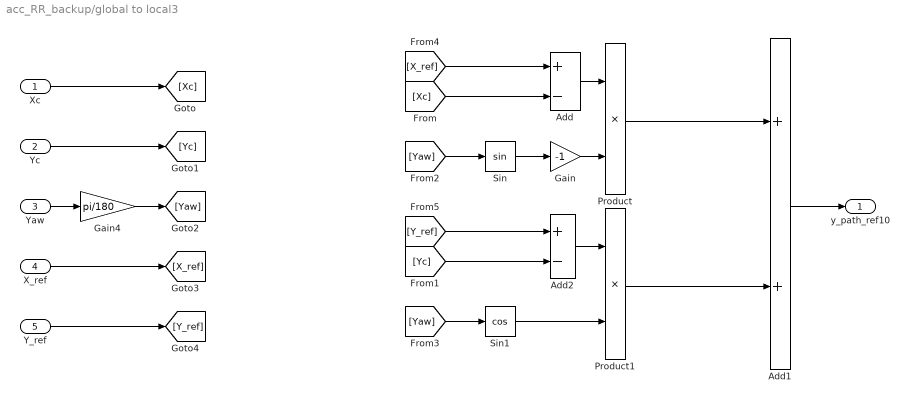
== system acc_RR_backup/global to local3 ==
  Xc : Inport
  Yc : Inport  Port=2
  Yaw : Inport  Port=3
  X_ref : Inport  Port=4
  Y_ref : Inport  Port=5
  Add : Sum  Inputs=+-
  Add1 : Sum
  Add2 : Sum  Inputs=+-
  Gain : Gain  Gain=-1
  Gain4 : Gain  Gain=pi/180
  Product : Product
  Product1 : Product
  Sin : Trigonometry
  Sin1 : Trigonometry  Operator=cos
  y_path_ref10 : Outport
  wires:
  Gain4/1 -> [Yaw]
  Y_ref/1 -> [Y_ref]
  X_ref/1 -> [X_ref]
  [Yaw] -> Sin1/1
  Yaw/1 -> Gain4/1
  Yc/1 -> [Yc]
  Xc/1 -> [Xc]
  [Xc] -> Add/2
  [Yc] -> Add2/2
  [Yaw] -> Sin/1
  Add1/1 -> y_path_ref10/1
  Product1/1 -> Add1/2
  Add2/1 -> Product1/1
  Sin1/1 -> Product1/2
  Product/1 -> Add1/1
  Add/1 -> Product/1
  Gain/1 -> Product/2
  Sin/1 -> Gain/1
  [Y_ref] -> Add2/1
  [X_ref] -> Add/1

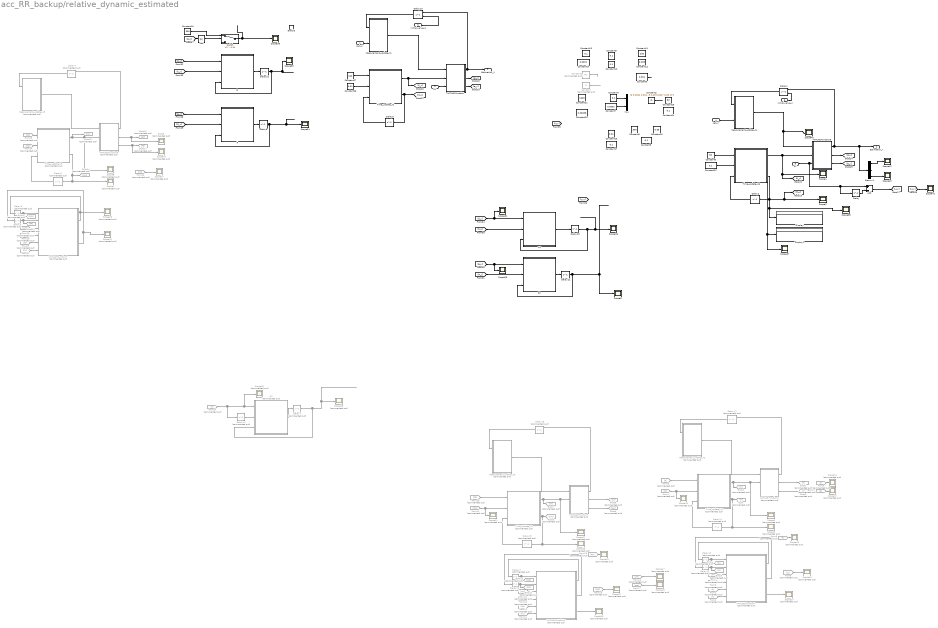
== system acc_RR_backup/relative_dynamic_estimated ==
  Jerk_X : Inport
  RX : Inport  Port=2
  Initial_value_X : Inport  Port=3
  Jerk_Y : Inport  Port=4
  RY : Inport  Port=5
  Initial_value_Y : Inport  Port=6
  Enable : EnablePort
  Abs : Abs
  Add : Sum  Inputs=+-
  Constant : Constant  Commented=on  Value=R
  Constant1 : Constant  Commented=on  Value=Rw
  Constant{4..5,9..10,13,17,22,24} (8 alike) : Constant  Value=0.1
  Constant11 : Constant  Value=200
  Constant12 : Constant  Value=0.005
  Constant14 : Constant  Value=0.0001
  Constant15 : Constant  Value=0.05
  Constant16 : Constant  Value=300
  Constant19 : Constant  Value=0.01
  Constant2 : Constant  Value=[0 0.0001 0.0017;0.0001 0.0025 0.05;0.0017 0.05 1]*1
  Constant20 : Constant  Value=0.00005
  Constant21 : Constant  Value=1000
  Constant25 : Constant  Value=50
  Constant26 : Constant  Value=0.01
  Constant27 : Constant  Value=100
  Constant3 : Constant  Value=0.001
  Constant6 : Constant  Value=50
  Constant7 : Constant  Value=0.0001
  Constant8 : Constant  Value=500
  Delay : Delay  DelayLength=1
  Delay1 : Delay  DelayLength=1  InitialConditionSource=Input port  InitialCondition=[0;0;0]  SampleTime=T
      settings: InputPortMap=u0,p4
  Delay10 : Delay  DelayLength=1  InitialConditionSource=Input port  InitialCondition=[0;0;0]  SampleTime=T
      settings: InputPortMap=u0,p4
  Delay11 : Delay  Commented=on  DelayLength=1  InitialConditionSource=Input port  InitialCondition=[0;0;0]  SampleTime=T
      settings: InputPortMap=u0,p4
  Delay12 : Delay  Commented=on  DelayLength=1  InitialCondition=[0 0 0;0 0 0.004;0 0.004 0.8]*0.001  SampleTime=T
  Delay13 : Delay  Commented=on  DelayLength=1  InitialCondition=0.001  SampleTime=T
  Delay14 : Delay  Commented=on  DelayLength=1  InitialCondition=[1 0 0;0 1 0;0 0 1]  SampleTime=T
  Delay15 : Delay  Commented=on  DelayLength=1  InitialConditionSource=Input port  InitialCondition=[0;0;0]  SampleTime=T
      settings: InputPortMap=u0,p4
  Delay16 : Delay  Commented=on  DelayLength=1  InitialCondition=0
  Delay17 : Delay  Commented=on  DelayLength=1  InitialCondition=[0 0 0;0 0 0.004;0 0.004 0.8]*0.01  SampleTime=T
  Delay18 : Delay  Commented=on  DelayLength=1  InitialCondition=0.001  SampleTime=T
  Delay19 : Delay  Commented=on  DelayLength=1  InitialCondition=[1 0 0;0 1 0;0 0 1]  SampleTime=T
  Delay2 : Delay  DelayLength=1  InitialCondition=[1 0 0;0 1 0;0 0 1]  SampleTime=T
  Delay21 : Delay  DelayLength=1  InitialCondition=[0 0.0001 0.0017;0.0001 0.0025 0.05;0.0017 0.05 1]
  Delay22 : Delay  DelayLength=1  InitialCondition=0.001
  Delay23 : Delay  DelayLength=1  InitialCondition=[0 0.0001 0.0017;0.0001 0.0025 0.05;0.0017 0.05 1]*1e-5
  Delay3 : Delay  Commented=on  DelayLength=1  InitialCondition=[0 0 0;0 0 0.003;0 0.003 0.005]  SampleTime=T
  Delay4 : Delay  Commented=on  DelayLength=1  InitialConditionSource=Input port  InitialCondition=[0;0;0]  SampleTime=T
      settings: InputPortMap=u0,p4
  Delay5 : Delay  Commented=on  DelayLength=1  InitialCondition=0.001  SampleTime=T
  Delay6 : Delay  Commented=on  DelayLength=1  InitialCondition=[1 0 0;0 1 0;0 0 1]  SampleTime=T
  Delay7 : Delay  Commented=on  DelayLength=1  InitialCondition=0.1
  Delay8 : Delay  DelayLength=1  InitialCondition=0.1
  Delay9 : Delay  DelayLength=1  InitialCondition=[1 0 0;0 1 0;0 0 1]  SampleTime=T
  Demux1 : Demux  Outputs=3
  Display : Display
  Display1 : Display
  From : From  Commented=on  GotoTag=M
  From1 : From  Commented=on  GotoTag=K
  From10 : From  Commented=on  GotoTag=MM
  From11 : From  Commented=on  GotoTag=KK
  From12 : From  Commented=on  GotoTag=dd
  From13 : From  Commented=on  GotoTag=ee
  From14 : From  Commented=on  GotoTag=QQ
  From15 : From  Commented=on  GotoTag=RR
  From16 : From  Commented=on  GotoTag=dd
  From17 : From  Commented=on  GotoTag=ee
  From18 : From  Commented=on  GotoTag=RR
  From19 : From  Commented=on  GotoTag=QQ
  From2 : From  Commented=on  GotoTag=d
  From20 : From  Commented=on  GotoTag=MM
  From21 : From  Commented=on  GotoTag=KK
  From22 : From  Commented=on  GotoTag=dd
  From23 : From  Commented=on  GotoTag=ee
  From24 : From  Commented=on  GotoTag=QQ
  From25 : From  Commented=on  GotoTag=RR
  From26 : From  Commented=on  GotoTag=KK
  From27 : From  Commented=on  GotoTag=d
  From3 : From  Commented=on  GotoTag=e
  From4 : From  Commented=on  GotoTag=Q
  From5 : From  Commented=on  GotoTag=R
  From6 : From  Commented=on  GotoTag=d
  From7 : From  Commented=on  GotoTag=e
  From8 : From  Commented=on  GotoTag=R
  From9 : From  Commented=on  GotoTag=Q
  Goto : Goto  Commented=on  GotoTag=M
  Goto1 : Goto  Commented=on  GotoTag=K
  Goto10 : Goto  Commented=on  GotoTag=QQ
  Goto11 : Goto  Commented=on  GotoTag=RR
  Goto12 : Goto  Commented=on  GotoTag=QQ
  Goto13 : Goto  Commented=on  GotoTag=RR
  Goto14 : Goto  Commented=on  GotoTag=MM
  Goto15 : Goto  Commented=on  GotoTag=KK
  Goto16 : Goto  Commented=on  GotoTag=dd
  Goto17 : Goto  Commented=on  GotoTag=ee
  Goto2 : Goto  Commented=on  GotoTag=d
  Goto3 : Goto  Commented=on  GotoTag=e
  Goto4 : Goto  Commented=on  GotoTag=Q
  Goto5 : Goto  Commented=on  GotoTag=R
  Goto6 : Goto  Commented=on  GotoTag=MM
  Goto7 : Goto  Commented=on  GotoTag=KK
  Goto8 : Goto  Commented=on  GotoTag=dd
  Goto9 : Goto  Commented=on  GotoTag=ee
  MATLAB Function : MATLAB Function  TreatAsAtomicUnit=on
  MATLAB Function1 : MATLAB Function  Commented=on  TreatAsAtomicUnit=on
  MATLAB Function2 : MATLAB Function  Commented=on  TreatAsAtomicUnit=on
  MATLAB Function3 : MATLAB Function  Commented=on  TreatAsAtomicUnit=on
  MATLAB Function4 : MATLAB Function  Commented=on  TreatAsAtomicUnit=on
  MATLAB Function5 : MATLAB Function  TreatAsAtomicUnit=on
  MATLAB Function6 : MATLAB Function  Commented=on  TreatAsAtomicUnit=on
  MATLAB Function7 : MATLAB Function  Commented=on  TreatAsAtomicUnit=on
  Measurement_update_X1 : MATLAB Function  TreatAsAtomicUnit=on
  Measurement_update_X2 : MATLAB Function  Commented=on  TreatAsAtomicUnit=on
  Measurement_update_X3 : MATLAB Function  Commented=on  TreatAsAtomicUnit=on
  Measurement_update_X4 : MATLAB Function  TreatAsAtomicUnit=on
  Measurement_update_X5 : MATLAB Function  Commented=on  TreatAsAtomicUnit=on
  Mux : Mux  Inputs=2
  Q : MATLAB Function  TreatAsAtomicUnit=on
  Q1 : MATLAB Function  Commented=on  TreatAsAtomicUnit=on
  Q2 : MATLAB Function  TreatAsAtomicUnit=on
  R : MATLAB Function  TreatAsAtomicUnit=on
  R2 : MATLAB Function  TreatAsAtomicUnit=on
  Scope{,6..28,30} (25 alike) : Scope  Commented=on
  Scope{1..2,5,29,31,34..43} (15 alike) : Scope
  Switch : Switch  Criteria=u2 > Threshold  Threshold=0.04
  Time_update_X1 : MATLAB Function  TreatAsAtomicUnit=on
  Time_update_X2 : MATLAB Function  Commented=on  TreatAsAtomicUnit=on
  Time_update_X3 : MATLAB Function  Commented=on  TreatAsAtomicUnit=on
  Time_update_X5 : MATLAB Function  Commented=on  TreatAsAtomicUnit=on
  Time_update_X6 : MATLAB Function  TreatAsAtomicUnit=on
  Estimation_X : Outport  VectorParamsAs1DForOutWhenUnconnected=off
  Estimation_Y : Outport  Port=2  VectorParamsAs1DForOutWhenUnconnected=off
  wires:
  MATLAB Function/3(e) -> [e_x]
  MATLAB Function/2(d) -> [d_x]
  Constant27/1 -> Time_update_X1/1(Q)
  Constant26/1 -> Time_update_X1/2(R)
  Abs/1 -> Switch/2
  [d_x] -> Abs/1
  Constant16/1 -> Switch/1
  Switch/1 -> Scope39/1
  Constant22/1 -> Time_update_X6/2(R)
  Constant6/1 -> Time_update_X6/1(Q)
  Demux1/3 -> Scope43/1
  Demux1/1 -> Scope42/1
  [yyy] -> Scope41/1
  Delay/1 -> Add/2
  Add/1 -> [yyy]
  Delay22/1 -> Scope5/1, R2/3(R1)
  Constant7/1 -> Mux/2
  Constant4/1 -> Mux/1
  Demux1/2 -> ?
  Delay23/1 -> Scope36/1, Q2/3(Q1)
  Time_update_X6/2(P) -> Display1/1, Scope37/1
  Constant3/1 -> ?
  Constant2/1 -> ?
  Q2/1(Q) -> Delay23/1
  Constant1/1 -> ?
  Constant/1 -> ?
  MATLAB Function5/3(e) -> [e_y]
  MATLAB Function5/2(d) -> [d_y]
  [d_y] -> Q2/1(d), Scope31/1
  [K_y] -> Q2/2(K)
  R2/1(R) -> Delay22/1
  [M_y] -> R2/2(M)
  [e_y] -> R2/1(e), Scope29/1
  Q1/1(Rw) -> Delay7/1
  From27/1 -> Q1/1(d), Scope30/1, Delay16/1
  Delay7/1 -> Scope28/1, Q1/3(Rw1)
  Delay16/1 -> Q1/2(dx)
  Delay21/1 -> Q/3(Q1), Scope35/1
  Q/1(Q) -> Delay21/1
  [K_x] -> Q/2(K)
  [d_x] -> Q/1(d)
  [M_x] -> R/2(M)
  R/1(R) -> Delay8/1
  [e_x] -> R/1(e)
  Delay8/1 -> R/3(R1), Scope34/1
  RX/1 -> MATLAB Function/3(y)
  From26/1 -> Scope27/1
  Initial_value_X/1 -> Delay10/2
  Delay4/1 -> Measurement_update_X5/1(X_e)
  MATLAB Function6/1(X_e) -> Delay4/1
  Measurement_update_X5/1(X_b) -> MATLAB Function6/1(X_b)
  Time_update_X5/2(M2) -> Scope7/1, Delay6/1, Goto14/1
  From22/1 -> MATLAB Function7/5(d)
  Delay6/1 -> Time_update_X5/3(M)
  Time_update_X5/1(K) -> MATLAB Function6/2(K), Scope6/1, Goto15/1
  From21/1 -> MATLAB Function7/6(K)
  From20/1 -> MATLAB Function7/3(M)
  MATLAB Function7/2(R2) -> Delay5/1, Scope26/1
  MATLAB Function6/3(e) -> Goto17/1, Scope24/1
  From24/1 -> Time_update_X5/2(Q)
  From25/1 -> Time_update_X5/1(R)
  MATLAB Function7/1(Q2) -> Scope25/1, Delay3/1
  From23/1 -> MATLAB Function7/4(e)
  Delay5/1 -> Goto13/1, MATLAB Function7/2(R)
  Delay3/1 -> Goto12/1, MATLAB Function7/1(Q)
  MATLAB Function6/2(d) -> Goto16/1, Scope/1
  RY/1 -> MATLAB Function5/3(y), Delay/1, Add/1
  Initial_value_Y/1 -> Delay1/2
  Measurement_update_X4/1(X_b) -> MATLAB Function5/1(X_b), Scope40/1
  MATLAB Function5/1(X_e) -> Delay1/1, Estimation_Y/1, Demux1/1
  Delay1/1 -> Measurement_update_X4/1(X_e)
  Time_update_X6/1(K) -> Scope1/1, [K_y], MATLAB Function5/2(K)
  Time_update_X6/3(M2) -> Delay2/1, Scope2/1, [M_y], Display/1, Scope38/1
  Delay2/1 -> Time_update_X6/3(M)
  Jerk_Y/1 -> Measurement_update_X4/2(u)
  Jerk_X/1 -> Measurement_update_X1/2(u)
  MATLAB Function3/2(d) -> Goto8/1
  Delay17/1 -> MATLAB Function4/1(Q), Goto10/1
  Time_update_X3/1(K) -> MATLAB Function3/2(K), Scope22/1, Goto7/1
  From13/1 -> MATLAB Function4/4(e)
  From15/1 -> Time_update_X3/1(R)
  From19/1 -> Scope21/1
  MATLAB Function4/1(Q2) -> Delay17/1
  Delay18/1 -> MATLAB Function4/2(R), Goto11/1
  From10/1 -> MATLAB Function4/3(M)
  MATLAB Function4/2(R2) -> Delay18/1
  Delay15/1 -> Measurement_update_X3/1(X_e)
  From11/1 -> MATLAB Function4/6(K)
  Delay19/1 -> Time_update_X3/3(M)
  From12/1 -> MATLAB Function4/5(d)
  From17/1 -> Scope18/1
  From18/1 -> Scope19/1
  From16/1 -> Scope17/1
  MATLAB Function3/3(e) -> Goto9/1
  Time_update_X3/2(M2) -> Goto6/1, Delay19/1, Scope23/1
  Measurement_update_X3/1(X_b) -> MATLAB Function3/1(X_b)
  From14/1 -> Time_update_X3/2(Q), Scope16/1
  MATLAB Function3/1(X_e) -> Delay15/1
  MATLAB Function4/3(G) -> Scope20/1
  From9/1 -> Scope15/1
  MATLAB Function2/3(G) -> Scope14/1
  From8/1 -> Scope13/1
  From7/1 -> Scope12/1
  From6/1 -> Scope11/1
  From4/1 -> Time_update_X2/2(Q), Scope10/1
  MATLAB Function2/1(Q2) -> Delay12/1
  Time_update_X2/2(M2) -> Goto/1, Delay14/1, Scope9/1
  From1/1 -> MATLAB Function2/6(K)
  Delay13/1 -> MATLAB Function2/2(R), Goto5/1
  Delay14/1 -> Time_update_X2/3(M)
  Time_update_X2/1(K) -> MATLAB Function1/2(K), Scope8/1, Goto1/1
  Delay11/1 -> Measurement_update_X2/1(X_e)
  Measurement_update_X2/1(X_b) -> MATLAB Function1/1(X_b)
  MATLAB Function1/1(X_e) -> Delay11/1
  MATLAB Function1/2(d) -> Goto2/1
  From2/1 -> MATLAB Function2/5(d)
  From5/1 -> Time_update_X2/1(R)
  MATLAB Function1/3(e) -> Goto3/1
  MATLAB Function2/2(R2) -> Delay13/1
  From/1 -> MATLAB Function2/3(M)
  From3/1 -> MATLAB Function2/4(e)
  Delay12/1 -> MATLAB Function2/1(Q), Goto4/1
  MATLAB Function/1(X_e) -> Delay10/1, Estimation_X/1
  Time_update_X1/2(M2) -> Delay9/1, [M_x]
  Measurement_update_X1/1(X_b) -> MATLAB Function/1(X_b)
  Delay9/1 -> Time_update_X1/3(M)
  Delay10/1 -> Measurement_update_X1/1(X_e)
  Time_update_X1/1(K) -> MATLAB Function/2(K), [K_x]
